simulink model "bike_model"  (R2022b)
settings: Solver=FixedStepAuto  StartTime=0.0  StopTime=inf  FixedStep=0.005  RelTol=1e-3
libraries: autolibshared x2
settings Model: Creator=LinF  LastModifiedBy=LinF
settings SolverCC: ConcurrentTasks=on  PositivePriorityOrder=on
settings OptimizationCC: BlockReduction=off  OptimizeBlockIOStorage=off
settings DebuggingCC: TasksWithSamePriorityMsg=none
settings HardwareCC: ProdBitPerLong=64  ProdLongLongMode=on  ProdHWDeviceType=Intel->x86-64 (Linux 64)
settings RTWCC: Description=Simulink Real-Time  SystemTargetFile=slrealtime.tlc  TemplateMakefile=slrealtime_default_tmf  Toolchain=Simulink Real-Time Toolchain  BuildConfiguration=Faster Runs  CodeExecutionProfiling=on  TargetLang=C++

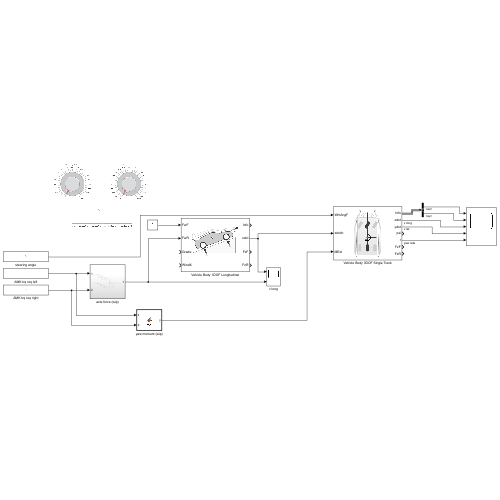
[thumbnail: Simulink's stored preview of the top-level diagram]
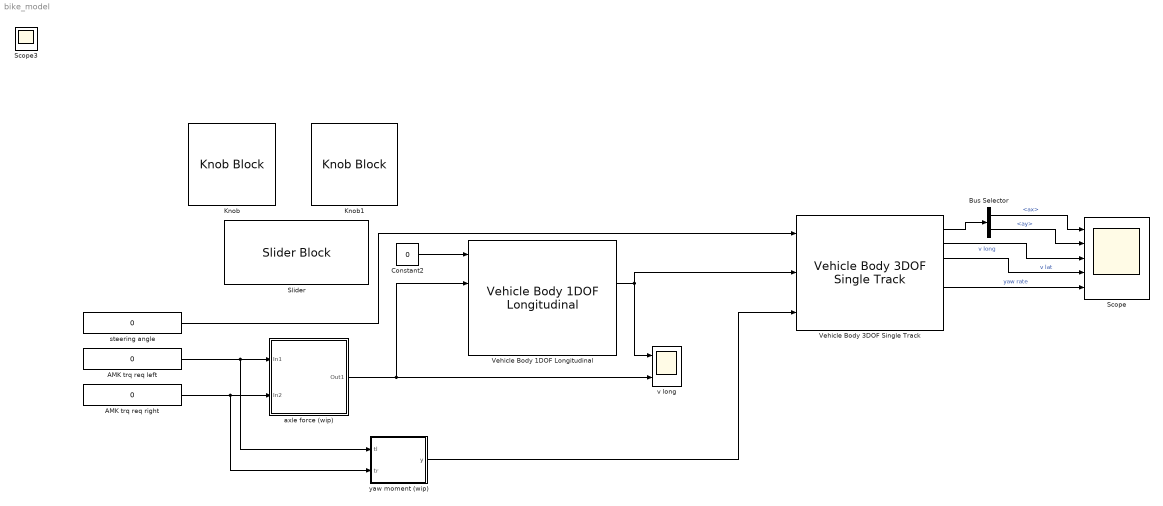
== system bike_model ==
  AMK trq req left : Constant  Value=0
  AMK trq req right : Constant  Value=0
  Bus Selector : BusSelector  OutputSignals=BdyFrm.Cg.Acc.ax,BdyFrm.Cg.Acc.ay
  Constant2 : Constant  Value=0
  Knob : KnobBlock  ScaleMax=1000
  Knob1 : KnobBlock  ScaleMax=1000
  Scope : Scope  NumInputPorts=5
  Slider : SliderBlock  ScaleMin=-1  ScaleMax=1
  Vehicle Body 1DOF Longitudinal : autolibshared/Vehicle Body 1DOF Longitudinal  VariantControl=SL  extFMode=off  extMMode=off  extTamb=off  wind3D=off  aMode=2  NF=2  NR=2  m=300  a=0.756  b=0.756  h=0.2  Cd=0  Cl=0  Cpm=0  Af=0  x_o=0  xdot_o=0  Pabs=101325  T=273  g=9.81
      settings: LibrarySourceBlock=vehdynlibeom/Vehicle Body 1DOF Longitudinal
  Vehicle Body 3DOF Single Track : autolibshared/Vehicle Body 3DOF Single Track  trackMode=Single (bicycle)  inputMode=External longitudinal velocity  frontSteerMode=on  rearSteerMode=off  windMode=off  muMode=off  extFMode=off  extMMode=on  htchFMode=off  htchMMode=off  extXo=off  extpsio=off  extxdoto=off  extro=off  extYo=off  extTamb=off  extydoto=off  aMode=2  NF=2  NR=2  m=300  a=0.756  b=0.756  h=0.2  dh=1  hh=0.2  X_o=0  xdot_o=0  CalphaMode=off  sigmaMode=off  d=0  hl=0  w=[1.4,1.4]  Cy_f=12e3  Cy_r=12e3  sigma_f=.1  sigma_r=.1  alpha_f_brk=[-.1 .1]  Cy_f_data=[-9e3 9e3]  alpha_r_brk=[-.1 .1]  Cy_r_data=[-9e3 9e3]  Y_o=0  ydot_o=0  Izz=4000  psi_o=0  r_o=0  Af=0  Cd=0  Cl=0  Cpm=.1  beta_w=[0 0.01:0.01:0.3]  Cs=[0 0.01:0.01:0.3]  Cym=[0 1e-6:0.01:0.3]  Pabs=101325  Tair=273  g=9.81  mu=1  xdot_tol=.01  Fznom=5000  Fxtire_sat=7e4  Fytire_sat=7e4  longOff=0  latOff=0  vertOff=0  wrapAng=off
  axle force (wip) : Subsystem
  steering angle : Constant  Value=0
  v long : Scope  NumInputPorts=2
  yaw moment (wip) : MATLAB Function  TreatAsAtomicUnit=on
  Scope3 : Scope
  wires:
  Constant2/1 -> Vehicle Body 1DOF Longitudinal/1
  steering angle/1 -> Vehicle Body 3DOF Single Track/1
  Vehicle Body 1DOF Longitudinal/2 -> Vehicle Body 3DOF Single Track/2, v long/1
  Vehicle Body 3DOF Single Track/1 -> Bus Selector/1
  Vehicle Body 3DOF Single Track/3 -> Scope/4  "v lat"
  Vehicle Body 3DOF Single Track/2 -> Scope/3  "v long"
  Vehicle Body 3DOF Single Track/5 -> Scope/5  "yaw rate"
  Bus Selector/1 -> Scope/1  "<ax>"
  Bus Selector/2 -> Scope/2  "<ay>"
  axle force (wip)/1(Out1) -> Vehicle Body 1DOF Longitudinal/2, v long/2
  AMK trq req left/1 -> yaw moment (wip)/1(tl), axle force (wip)/1(In1)
  yaw moment (wip)/1(y) -> Vehicle Body 3DOF Single Track/3
  AMK trq req right/1 -> yaw moment (wip)/2(tr), axle force (wip)/2(In2)

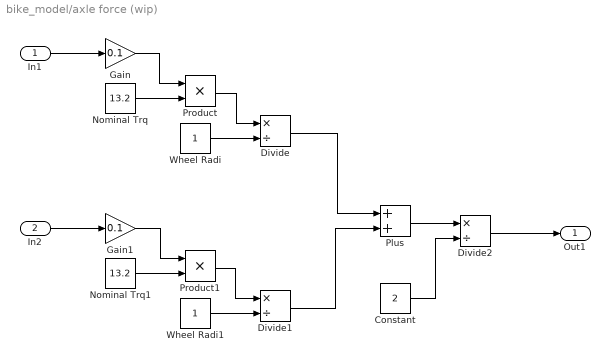
== system bike_model/axle force (wip) ==
  In1 : Inport
  In2 : Inport  Port=2
  Constant : Constant  Value=2
  Divide : Product  Inputs=*/
  Divide1 : Product  Inputs=*/
  Divide2 : Product  Inputs=*/
  Gain : Gain  Gain=0.1
  Gain1 : Gain  Gain=0.1
  Nominal Trq : Constant  Value=13.2
  Nominal Trq1 : Constant  Value=13.2
  Plus : Sum
  Product : Product
  Product1 : Product
  Wheel Radi : Constant
  Wheel Radi1 : Constant
  Out1 : Outport
  wires:
  Wheel Radi/1 -> Divide/2
  Gain/1 -> Product/1
  Nominal Trq/1 -> Product/2
  In1/1 -> Gain/1
  Divide/1 -> Plus/1
  Product/1 -> Divide/1
  Gain1/1 -> Product1/1
  Wheel Radi1/1 -> Divide1/2
  Product1/1 -> Divide1/1
  In2/1 -> Gain1/1
  Nominal Trq1/1 -> Product1/2
  Divide1/1 -> Plus/2
  Plus/1 -> Divide2/1
  Constant/1 -> Divide2/2
  Divide2/1 -> Out1/1

== matlab function bike_model/yaw moment (wip) ==
  data: tl input; y output; tr input
function y = fcn(tl,tr)
m = tl-tr;
y = [0,0,m];
